simulink model "Sim5_MMC"  (R2017b)
settings: Solver=ode1  StartTime=0.0  StopTime=4  FixedStep=Time_Step  RelTol=1e-3
undefined symbols (not defined in the file): DiscIntNeverNeededParam, GRD00_Lg, GRD00_Rg, Time_Step, VSC01_id0
libraries: powerlib x107, Control_Lib x16, simulink x15, spsCurrentMeasurementLib x14, powerlib_meascontrol x4
(part 2 of 5)

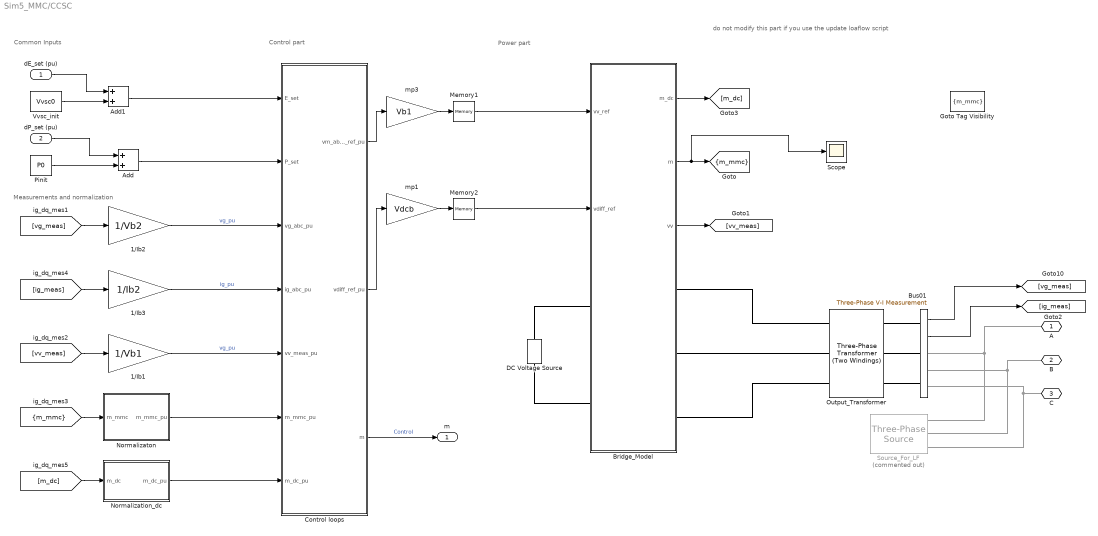
== system Sim5_MMC/CCSC ==
  note: do not modify this part if you use the update loaflow script
  note: Common Inputs
  note: Power part
  note: Measurements and normalization
  note: Control part
  dE_set (pu) : Inport
  dP_set (pu) : Inport  Port=2
  1/Ib1 : Gain  Gain=1/Vb1
  1/Ib2 : Gain  Gain=1/Vb2
  1/Ib3 : Gain  Gain=1/Ib2
  Add : Sum
  Add1 : Sum
  Bridge_Model : Subsystem
  Bus01 : powerlib/Measurements/Three-Phase V-I Measurement  VoltageMeasurement=phase-to-ground  SetLabelV=off  LabelV=Vabc  Vpu=off  VpuLL=off  CurrentMeasurement=yes  SetLabelI=off  LabelI=Iabc  Ipu=off  Pbase=100e6  Vbase=500e3  OutputType=Complex  PhasorSimulation=off  PSBequivalent=0
  Control loops : Subsystem
  DC Voltage Source : powerlib/Electrical Sources/DC Voltage Source  Amplitude=Udcn  Measurements=Voltage
  Goto Tag Visibility : GotoTagVisibility  GotoTag=m_mmc
  Memory1 : Memory  InitialCondition=[Va0 Vb0 Vc0]
  Memory2 : Memory  InitialCondition=[Udcn/2 Udcn/2 Udcn/2]
  Normalization_dc : Subsystem
  Normalizaton : Subsystem
  Output_Transformer : powerlib/Elements/Three-Phase Transformer (Two Windings)  Winding1Connection=Yg  Winding2Connection=Yg  CoreType=Three single-phase transformers  SetSaturation=off  Hysteresis=off  DataFile='hysteresis'  SetInitialFlux=off  Measurements=None  UNITS=pu  NominalPower=[Sn , fb]  Winding1=[Un1 , Rt_pu/2 , Lt_pu/2]  Winding2=[Un2 , Rt_pu/2 , Lt_pu/2]  Rm=Rm_pu  Lm=Lm_pu  L0=0.5  Saturation=[ 0,0 ; 0.0024,1.2 ; 1.0,1.52 ]  InitialFluxes=[ 0.8 , -0.8 , 0.7 ]  BreakLoop=off  DiscreteSolver=Trapezoidal iterative  DataType=off  TransfoNumber=1
  Pinit : Constant  Value=P0
  Scope : Scope
  Source_For_LF : powerlib/Electrical Sources/Three-Phase Source  Commented=on  InternalConnection=Yg  VoltagePhases=off  Voltage=(400000)*1.00095  PhaseAngle=0.57242  Voltage_phases=[25e3 25e3 25e3]/sqrt(3)  PhaseAngles_phases=[0 -120 +120]  Frequency=fb  NonIdealSource=off  SpecifyImpedance=off  Resistance=0  Inductance=0  ShortCircuitLevel=100e6  BaseVoltage=Un  XRratio=7  BusType=PQ  Pref=P0*Sb  Qref=Q0*Sb  Prefabc=[10e3, 10e3, 10e3]  Qrefabc=[0, 0, 0]  Qmin=-inf  Qmax=inf
  Vvsc_init : Constant  Value=Vvsc0
  mp1 : Gain  Gain=Vdcb
  mp3 : Gain  Gain=Vb1
  A : PMIOPort  Side=Right
  B : PMIOPort  Port=2  Side=Right
  C : PMIOPort  Port=3  Side=Right
  m : Outport  VectorParamsAs1DForOutWhenUnconnected=off
  tag scope: m_mmc=scoped
  wires:
  Add/1 -> Control loops/2(P_set)
  Control loops/3(m) -> m/1  "Control"
  mp3/1 -> Memory1/1
  1/Ib3/1 -> Control loops/4(ig_abc_pu)  "ig_pu"
  1/Ib2/1 -> Control loops/3(vg_abc_pu)  "vg_pu"
  [vg_meas] -> 1/Ib2/1
  Control loops/1(vm_abc_ref_pu) -> mp3/1
  Add1/1 -> Control loops/1(E_set)
  Memory1/1 -> Bridge_Model/1(vv_ref)
  dP_set (pu)/1 -> Add/1
  Pinit/1 -> Add/2
  Vvsc_init/1 -> Add1/2
  Bus01/1 -> [vg_meas]
  dE_set (pu)/1 -> Add1/1
  Bus01/2 -> [ig_meas]
  [ig_meas] -> 1/Ib3/1
  Control loops/2(vdiff_ref_pu) -> mp1/1
  mp1/1 -> Memory2/1
  Memory2/1 -> Bridge_Model/2(vdiff_ref)
  Bridge_Model/3(vv) -> [vv_meas]
  [vv_meas] -> 1/Ib1/1
  1/Ib1/1 -> Control loops/5(vv_meas_pu)  "vg_pu"
  [m_mmc] -> Normalizaton/1(m_mmc)
  Normalizaton/1(m_mmc_pu) -> Control loops/6(m_mmc_pu)
  Bridge_Model/1(m_dc) -> [m_dc]
  Normalization_dc/1(m_dc_pu) -> Control loops/7(m_dc_pu)
  [m_dc] -> Normalization_dc/1(m_dc)
  Bridge_Model/2(m) -> Scope/1, [m_mmc]
  connections:
  DC Voltage Source/LConn1 -- Bridge_Model/LConn2
  Output_Transformer/RConn1 -- Bus01/LConn1
  Output_Transformer/RConn2 -- Bus01/LConn2
  DC Voltage Source/RConn1 -- Bridge_Model/LConn1
  Output_Transformer/RConn3 -- Bus01/LConn3
  Source_For_LF/RConn2 -- B/RConn1 -- Bus01/RConn2
  Source_For_LF/RConn1 -- A/RConn1 -- Bus01/RConn1
  Source_For_LF/RConn3 -- C/RConn1 -- Bus01/RConn3
  Bridge_Model/RConn1 -- Output_Transformer/LConn1
  Bridge_Model/RConn2 -- Output_Transformer/LConn2
  Bridge_Model/RConn3 -- Output_Transformer/LConn3

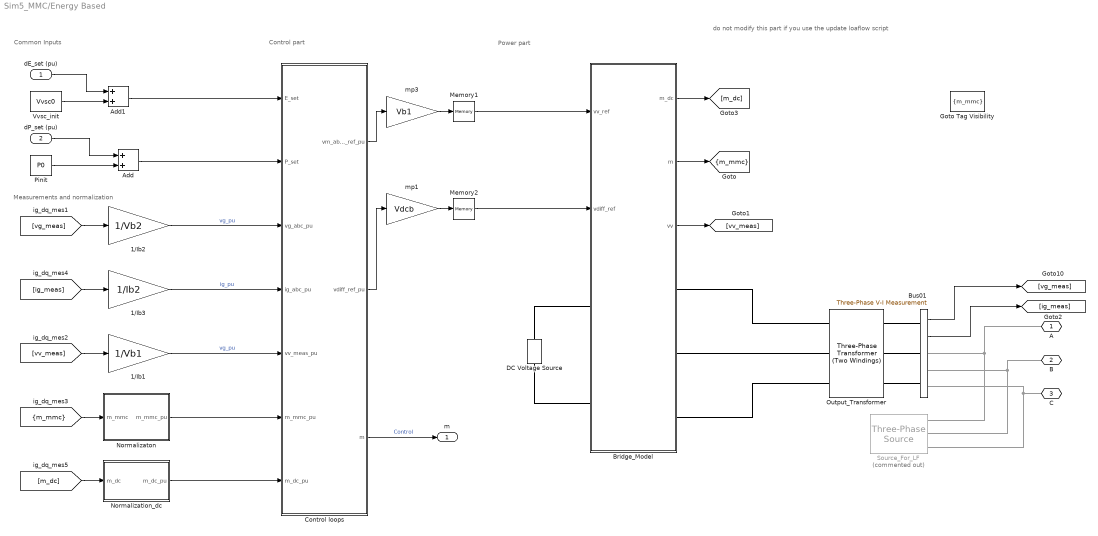
== system Sim5_MMC/Energy Based ==
  note: do not modify this part if you use the update loaflow script
  note: Common Inputs
  note: Power part
  note: Measurements and normalization
  note: Control part
  dE_set (pu) : Inport
  dP_set (pu) : Inport  Port=2
  1/Ib1 : Gain  Gain=1/Vb1
  1/Ib2 : Gain  Gain=1/Vb2
  1/Ib3 : Gain  Gain=1/Ib2
  Add : Sum
  Add1 : Sum
  Bridge_Model : Subsystem
  Bus01 : powerlib/Measurements/Three-Phase V-I Measurement  VoltageMeasurement=phase-to-ground  SetLabelV=off  LabelV=Vabc  Vpu=off  VpuLL=off  CurrentMeasurement=yes  SetLabelI=off  LabelI=Iabc  Ipu=off  Pbase=100e6  Vbase=500e3  OutputType=Complex  PhasorSimulation=off  PSBequivalent=0
  Control loops : Subsystem
  DC Voltage Source : powerlib/Electrical Sources/DC Voltage Source  Amplitude=Udcn  Measurements=Voltage
  Goto Tag Visibility : GotoTagVisibility  GotoTag=m_mmc
  Memory1 : Memory  InitialCondition=[Va0 Vb0 Vc0]
  Memory2 : Memory  InitialCondition=[Udcn/2 Udcn/2 Udcn/2]
  Normalization_dc : Subsystem
  Normalizaton : Subsystem
  Output_Transformer : powerlib/Elements/Three-Phase Transformer (Two Windings)  Winding1Connection=Yg  Winding2Connection=Yg  CoreType=Three single-phase transformers  SetSaturation=off  Hysteresis=off  DataFile='hysteresis'  SetInitialFlux=off  Measurements=None  UNITS=pu  NominalPower=[Sn , fb]  Winding1=[Un1 , Rt_pu/2 , Lt_pu/2]  Winding2=[Un2 , Rt_pu/2 , Lt_pu/2]  Rm=Rm_pu  Lm=Lm_pu  L0=0.5  Saturation=[ 0,0 ; 0.0024,1.2 ; 1.0,1.52 ]  InitialFluxes=[ 0.8 , -0.8 , 0.7 ]  BreakLoop=off  DiscreteSolver=Trapezoidal iterative  DataType=off  TransfoNumber=1
  Pinit : Constant  Value=P0
  Source_For_LF : powerlib/Electrical Sources/Three-Phase Source  Commented=on  InternalConnection=Yg  VoltagePhases=off  Voltage=(400000)*1.00095  PhaseAngle=0.57242  Voltage_phases=[25e3 25e3 25e3]/sqrt(3)  PhaseAngles_phases=[0 -120 +120]  Frequency=fb  NonIdealSource=off  SpecifyImpedance=off  Resistance=0  Inductance=0  ShortCircuitLevel=100e6  BaseVoltage=Un  XRratio=7  BusType=PQ  Pref=P0*Sb  Qref=Q0*Sb  Prefabc=[10e3, 10e3, 10e3]  Qrefabc=[0, 0, 0]  Qmin=-inf  Qmax=inf
  Vvsc_init : Constant  Value=Vvsc0
  mp1 : Gain  Gain=Vdcb
  mp3 : Gain  Gain=Vb1
  A : PMIOPort  Side=Right
  B : PMIOPort  Port=2  Side=Right
  C : PMIOPort  Port=3  Side=Right
  m : Outport  VectorParamsAs1DForOutWhenUnconnected=off
  tag scope: m_mmc=scoped
  wires:
  Add/1 -> Control loops/2(P_set)
  Control loops/3(m) -> m/1  "Control"
  mp3/1 -> Memory1/1
  1/Ib3/1 -> Control loops/4(ig_abc_pu)  "ig_pu"
  1/Ib2/1 -> Control loops/3(vg_abc_pu)  "vg_pu"
  [vg_meas] -> 1/Ib2/1
  Control loops/1(vm_abc_ref_pu) -> mp3/1
  Add1/1 -> Control loops/1(E_set)
  Memory1/1 -> Bridge_Model/1(vv_ref)
  dP_set (pu)/1 -> Add/1
  Pinit/1 -> Add/2
  Vvsc_init/1 -> Add1/2
  Bus01/1 -> [vg_meas]
  dE_set (pu)/1 -> Add1/1
  Bus01/2 -> [ig_meas]
  [ig_meas] -> 1/Ib3/1
  Control loops/2(vdiff_ref_pu) -> mp1/1
  mp1/1 -> Memory2/1
  Memory2/1 -> Bridge_Model/2(vdiff_ref)
  Bridge_Model/3(vv) -> [vv_meas]
  [vv_meas] -> 1/Ib1/1
  1/Ib1/1 -> Control loops/5(vv_meas_pu)  "vg_pu"
  [m_mmc] -> Normalizaton/1(m_mmc)
  Normalizaton/1(m_mmc_pu) -> Control loops/6(m_mmc_pu)
  Bridge_Model/1(m_dc) -> [m_dc]
  Normalization_dc/1(m_dc_pu) -> Control loops/7(m_dc_pu)
  [m_dc] -> Normalization_dc/1(m_dc)
  Bridge_Model/2(m) -> [m_mmc]
  connections:
  DC Voltage Source/LConn1 -- Bridge_Model/LConn2
  Output_Transformer/RConn1 -- Bus01/LConn1
  Output_Transformer/RConn2 -- Bus01/LConn2
  DC Voltage Source/RConn1 -- Bridge_Model/LConn1
  Output_Transformer/RConn3 -- Bus01/LConn3
  Source_For_LF/RConn2 -- B/RConn1 -- Bus01/RConn2
  Source_For_LF/RConn1 -- A/RConn1 -- Bus01/RConn1
  Source_For_LF/RConn3 -- C/RConn1 -- Bus01/RConn3
  Bridge_Model/RConn1 -- Output_Transformer/LConn1
  Bridge_Model/RConn2 -- Output_Transformer/LConn2
  Bridge_Model/RConn3 -- Output_Transformer/LConn3

== system Sim5_MMC/Mean Model 2-Level L-filter ==
  note: do not modify this part if you use the update loaflow script
  note: Common Inputs
  note: Power part
  note: Measurements and normalization
  note: Control part
  dE_set (pu) : Inport
  dP_set (pu) : Inport  Port=2
  1/Ib2 : Gain  Gain=1/Vb2
  1/Ib3 : Gain  Gain=1/Ib2
  Add : Sum
  Add1 : Sum
  Bridge_Model : Subsystem
  Bus01 : powerlib/Measurements/Three-Phase V-I Measurement  VoltageMeasurement=phase-to-ground  SetLabelV=off  LabelV=Vabc  Vpu=off  VpuLL=off  CurrentMeasurement=yes  SetLabelI=off  LabelI=Iabc  Ipu=off  Pbase=100e6  Vbase=500e3  OutputType=Complex  PhasorSimulation=off  PSBequivalent=0
  Control loops : Subsystem
  DC Voltage Source : powerlib/Electrical Sources/DC Voltage Source  Amplitude=Udcn  Measurements=Voltage
  Memory1 : Memory  InitialCondition=[Va0 Vb0 Vc0]
  Output_Transformer : powerlib/Elements/Three-Phase Transformer (Two Windings)  Winding1Connection=Yg  Winding2Connection=Yg  CoreType=Three single-phase transformers  SetSaturation=off  Hysteresis=off  DataFile='hysteresis'  SetInitialFlux=off  Measurements=None  UNITS=pu  NominalPower=[Sn , fb]  Winding1=[Un1 , Rt_pu/2 , Lt_pu/2]  Winding2=[Un2 , Rt_pu/2 , Lt_pu/2]  Rm=Rm_pu  Lm=Lm_pu  L0=0.5  Saturation=[ 0,0 ; 0.0024,1.2 ; 1.0,1.52 ]  InitialFluxes=[ 0.8 , -0.8 , 0.7 ]  BreakLoop=off  DiscreteSolver=Trapezoidal iterative  DataType=off  TransfoNumber=1
  Pinit : Constant  Value=P0
  Source_For_LF : powerlib/Electrical Sources/Three-Phase Source  Commented=on  InternalConnection=Yg  VoltagePhases=off  Voltage=(400000)*1.00139  PhaseAngle=0.85782  Voltage_phases=[25e3 25e3 25e3]/sqrt(3)  PhaseAngles_phases=[0 -120 +120]  Frequency=fb  NonIdealSource=off  SpecifyImpedance=off  Resistance=0  Inductance=0  ShortCircuitLevel=100e6  BaseVoltage=Un  XRratio=7  BusType=PQ  Pref=P0*Sb  Qref=Q0*Sb  Prefabc=[10e3, 10e3, 10e3]  Qrefabc=[0, 0, 0]  Qmin=-inf  Qmax=inf
  Vvsc_init : Constant  Value=Vvsc0
  mp3 : Gain  Gain=Vb1
  A : PMIOPort  Side=Right
  B : PMIOPort  Port=2  Side=Right
  C : PMIOPort  Port=3  Side=Right
  m : Outport  VectorParamsAs1DForOutWhenUnconnected=off
  wires:
  Add/1 -> Control loops/2(P_set)
  Control loops/2(m) -> m/1  "Control"
  mp3/1 -> Memory1/1
  1/Ib3/1 -> Control loops/4(ig_abc_pu)  "ig_pu"
  1/Ib2/1 -> Control loops/3(vg_abc_pu)  "vg_pu"
  [vg_meas] -> 1/Ib2/1
  Control loops/1(vm_abc_ref_pu) -> mp3/1
  Add1/1 -> Control loops/1(E_set)
  Memory1/1 -> Bridge_Model/1(Uref)
  dP_set (pu)/1 -> Add/1
  Pinit/1 -> Add/2
  Vvsc_init/1 -> Add1/2
  Bus01/1 -> [vg_meas]
  dE_set (pu)/1 -> Add1/1
  Bus01/2 -> [ig_meas]
  [ig_meas] -> 1/Ib3/1
  connections:
  DC Voltage Source/LConn1 -- Bridge_Model/LConn2
  Output_Transformer/RConn1 -- Bus01/LConn1
  Output_Transformer/RConn2 -- Bus01/LConn2
  DC Voltage Source/RConn1 -- Bridge_Model/LConn1
  Output_Transformer/RConn3 -- Bus01/LConn3
  Source_For_LF/RConn2 -- B/RConn1 -- Bus01/RConn2
  Bridge_Model/RConn1 -- Output_Transformer/LConn1
  Bridge_Model/RConn2 -- Output_Transformer/LConn2
  Bridge_Model/RConn3 -- Output_Transformer/LConn3
  Source_For_LF/RConn1 -- A/RConn1 -- Bus01/RConn1
  Source_For_LF/RConn3 -- C/RConn1 -- Bus01/RConn3

== system Sim5_MMC/Subsystem2 ==

== system Sim5_MMC/CCSC/Bridge_Model ==
  vv_ref : Inport
  vdiff_ref : Inport  Port=2
  Bus1 : powerlib/Measurements/Three-Phase V-I Measurement  VoltageMeasurement=phase-to-ground  SetLabelV=off  LabelV=Vabc  Vpu=off  VpuLL=off  CurrentMeasurement=no  SetLabelI=off  LabelI=Iabc  Ipu=off  Pbase=100e6  Vbase=500e3  OutputType=Complex  PhasorSimulation=off  PSBequivalent=0
  Constant : Constant
  Current Measurement : spsCurrentMeasurementLib/Current Measurement  PhasorSimulation=off  OutputType=Complex  PSBequivalent=0
  Decoupling voltage : Subsystem
  MMC Average Model : Subsystem
  Memory : Memory
  Memory1 : Memory  InitialCondition=Udcn
  Modulation Index Generation : Subsystem
  Mux : Mux  Inputs=2
  NOT1 : Logic  Operator=NOT  IconShape=distinctive  AllPortsSameDT=off  OutDataTypeStr=boolean
  Three-Phase Breaker1 : powerlib/Elements/Three-Phase Breaker  InitialState=closed  SwitchA=on  SwitchB=on  SwitchC=on  SwitchTimes="[4/60  10/60]"  External=on  BreakerResistance=0.001  SnubberResistance=1e6  SnubberCapacitance=inf  Measurements=None
  Three-Phase Breaker2 : powerlib/Elements/Three-Phase Breaker  InitialState=open  SwitchA=on  SwitchB=on  SwitchC=on  SwitchTimes="[4/60  10/60]"  External=on  BreakerResistance=0.001  SnubberResistance=1e6  SnubberCapacitance=inf  Measurements=None
  Three-Phase Source : powerlib/Electrical Sources/Three-Phase Source  InternalConnection=Yg  VoltagePhases=off  Voltage=Vvsc0*Un1  PhaseAngle=Theta_vsc0  Voltage_phases=[25e3 25e3 25e3]/sqrt(3)  PhaseAngles_phases=[0 -120 +120]  Frequency=fb  NonIdealSource=off  SpecifyImpedance=off  Resistance=0  Inductance=0  ShortCircuitLevel=100e6  BaseVoltage=VSC01_Un1  XRratio=7  BusType=swing  Pref=0.3  Qref=0  Prefabc=[10e3, 10e3, 10e3]  Qrefabc=[0, 0, 0]  Qmin=-Inf  Qmax=Inf
  Voltage Measurement : powerlib/Measurements/Voltage Measurement  PhasorSimulation=off  OutputType=Complex  PSBequivalent=0
  PhA : PMIOPort  Side=Right
  PhB : PMIOPort  Port=2  Side=Right
  PhC : PMIOPort  Port=3  Side=Right
  Vdc+ : PMIOPort  Port=4  Side=Left
  Vdc- : PMIOPort  Port=5  Side=Left
  m_dc : Outport
  m : Outport  Port=2
  vv : Outport  Port=3
  wires:
  Constant/1 -> Memory/1
  NOT1/1 -> Three-Phase Breaker1/1
  Memory/1 -> NOT1/1, Three-Phase Breaker2/1
  vv_ref/1 -> Decoupling voltage/1(Vv_ref)
  vdiff_ref/1 -> Decoupling voltage/2(Vdiff_ref)
  Decoupling voltage/1(Vmu_ref) -> Modulation Index Generation/1(vmu_ref)
  Decoupling voltage/2(Vml_ref) -> Modulation Index Generation/2(vml_ref)
  MMC Average Model/1(m) -> m/1
  Voltage Measurement/1 -> Memory1/1  "Vdc"
  Current Measurement/1 -> Mux/2  "Idc"
  Mux/1 -> m_dc/1
  Modulation Index Generation/1(mul) -> MMC Average Model/1(mul)
  Bus1/1 -> vv/1
  Memory1/1 -> Mux/1
  connections:
  Three-Phase Breaker1/LConn1 -- Bus1/LConn1 -- Three-Phase Breaker2/LConn1
  Three-Phase Breaker1/LConn2 -- Bus1/LConn2 -- Three-Phase Breaker2/LConn2
  Three-Phase Breaker1/LConn3 -- Bus1/LConn3 -- Three-Phase Breaker2/LConn3
  MMC Average Model/LConn1 -- Three-Phase Breaker2/RConn1
  MMC Average Model/LConn2 -- Three-Phase Breaker2/RConn2
  MMC Average Model/LConn3 -- Three-Phase Breaker2/RConn3
  Three-Phase Source/RConn1 -- Three-Phase Breaker1/RConn1
  Three-Phase Source/RConn2 -- Three-Phase Breaker1/RConn2
  Three-Phase Source/RConn3 -- Three-Phase Breaker1/RConn3
  MMC Average Model/RConn1 -- Current Measurement/RConn1 -- Voltage Measurement/LConn1
  MMC Average Model/RConn2 -- Voltage Measurement/LConn2 -- Vdc-/RConn1
  Current Measurement/LConn1 -- Vdc+/RConn1
  PhB/RConn1 -- Bus1/RConn2
  PhC/RConn1 -- Bus1/RConn3
  PhA/RConn1 -- Bus1/RConn1

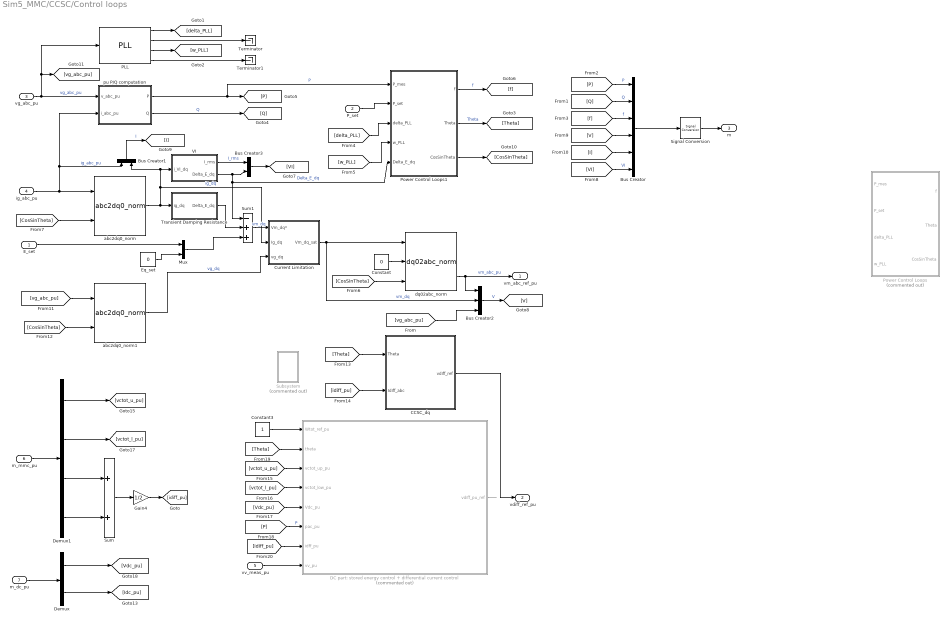
== system Sim5_MMC/CCSC/Control loops ==
  E_set : Inport
  P_set : Inport  Port=2
  vg_abc_pu : Inport  Port=3
  ig_abc_pu : Inport  Port=4
  vv_meas_pu : Inport  Port=5
  m_mmc_pu : Inport  Port=6
  m_dc_pu : Inport  Port=7
  " pu P/Q computation" : Subsystem  DialogController=POWERSYS.PowerSysDialog
  Bus Creator : BusCreator  Inputs=6
  Bus Creator1 : BusCreator  Inputs=2
  Bus Creator2 : BusCreator  Inputs=3
  Bus Creator3 : BusCreator  Inputs=2
  CCSC_dq : Subsystem
  Constant : Constant  Value=0
  Constant3 : Constant
  Current Limitation : Subsystem
  DC part: stored energy control + differential current control : Subsystem  Commented=on
  Demux : Demux  Outputs=2
  Demux1 : Demux  Outputs=[3 3 3 3]
  Eq_set : Constant  Value=0
  Gain4 : Gain  Gain=1/2
  Mux : Mux  Inputs=2
  PLL : Control_Lib/PLL  fb=fb  Tr_PLL=Tr_PLL  Theta0=Theta0
      settings: SourceProductName=VSC_Lib
  Power Control Loops : Subsystem  Commented=on
  Power Control Loops1 : Subsystem
  Signal Conversion : SignalConversion  OverrideOpt=off
  Subsystem : Subsystem  Commented=on
  Sum : Sum
  Sum1 : Sum  Inputs=-++
  Terminator : Terminator
  Terminator1 : Terminator
  Transient Damping Resistance : Subsystem
  VI : Subsystem
  abc2dq0_norm : Control_Lib/abc2dq0_norm  referenceAxisMode=Reference axis at 90 degrees behind phase_a  baseUpdateGain=1/sqrt(3)
      settings: SourceProductName=VSC_Lib
  abc2dq0_norm1 : Control_Lib/abc2dq0_norm  referenceAxisMode=Reference axis at 90 degrees behind phase_a  baseUpdateGain=1/sqrt(3)
      settings: SourceProductName=VSC_Lib
  dq02abc_norm : Control_Lib/dq02abc_norm  referenceAxisMode=Reference axis at 90 degrees behind phase_a  baseUpdateGain=sqrt(3)
      settings: SourceProductName=VSC_Lib
  vm_abc_ref_pu : Outport  VectorParamsAs1DForOutWhenUnconnected=off
  vdiff_ref_pu : Outport  Port=2
  m : Outport  Port=3  VectorParamsAs1DForOutWhenUnconnected=off
  wires:
  [vg_abc_pu] -> Bus Creator2/3
  Bus Creator3/1 -> [VI]
  PLL/4 -> Terminator1/1
  PLL/2 -> Terminator/1
  PLL/1 -> [delta_PLL]
  Constant/1 -> dq02abc_norm/2
  Power Control Loops1/3(CosSinTheta) -> [CosSinTheta]
  PLL/3 -> [w_PLL]
  [I] -> Bus Creator/5
  Bus Creator1/1 -> [I]  "I"
  Bus Creator/1 -> Signal Conversion/1
  [VI] -> Bus Creator/6  "VI"
  [V] -> Bus Creator/4
  Bus Creator2/1 -> [V]  "V"
  Eq_set/1 -> Mux/2
  Mux/1 -> Sum1/3
  VI/1(I_rms) -> Bus Creator3/1  "I_rms"
  Transient Damping Resistance/1("Delta_E_dq ") -> Sum1/2
  VI/2(Delta_E_dq) -> Power Control Loops1/5(Delta_E_dq), Sum1/1, Bus Creator3/2  "Delta_E_dq"
  [CosSinTheta] -> abc2dq0_norm/2
  [CosSinTheta] -> dq02abc_norm/3
  Power Control Loops1/2(Theta) -> [Theta]  "Theta"
  abc2dq0_norm/2 -> Bus Creator1/2, VI/1(i_VI_dq), Current Limitation/2(Ig_dq), Transient Damping Resistance/1(ig_dq)  "ig_dq"
  ig_abc_pu/1 -> abc2dq0_norm/1, " pu P/Q computation"/2(i_abc_pu), Bus Creator1/1  "ig_abc_pu"
  " pu P/Q computation"/1(P) -> Power Control Loops1/1(P_mes), [P]  "P"
  vg_abc_pu/1 -> PLL/1, [vg_abc_pu], " pu P/Q computation"/1(v_abc_pu)  "vg_abc_pu"
  Power Control Loops1/1(f) -> [f]  "f"
  [w_PLL] -> Power Control Loops1/4(w_PLL)
  P_set/1 -> Power Control Loops1/2(P_set)
  [delta_PLL] -> Power Control Loops1/3(delta_PLL)
  Current Limitation/1(Vm_dq_sat) -> dq02abc_norm/1, Bus Creator2/2  "vm_dq"
  " pu P/Q computation"/2(Q) -> [Q]  "Q"
  E_set/1 -> Mux/1
  dq02abc_norm/2 -> vm_abc_ref_pu/1, Bus Creator2/1  "vm_abc_pu"
  [f] -> Bus Creator/3  "f"
  [Q] -> Bus Creator/2  "Q"
  [P] -> Bus Creator/1  "P"
  Signal Conversion/1 -> m/1
  Sum1/1 -> Current Limitation/1(Vm_dq*)  "vm_dq"
  [vg_abc_pu] -> abc2dq0_norm1/1
  [CosSinTheta] -> abc2dq0_norm1/2
  abc2dq0_norm1/2 -> Current Limitation/3(vg_dq)  "vg_dq"
  [idiff_pu] -> CCSC_dq/2(Idiff_abc)
  CCSC_dq/1(vdiff_ref) -> vdiff_ref_pu/1
  Demux1/2 -> [vctot_l_pu]
  Demux1/1 -> [vctot_u_pu]
  m_mmc_pu/1 -> Demux1/1
  Demux/2 -> [Idc_pu]
  Demux/1 -> [Vdc_pu]
  m_dc_pu/1 -> Demux/1
  [Theta] -> CCSC_dq/1(Theta)
  Gain4/1 -> [idiff_pu]
  Sum/1 -> Gain4/1
  Demux1/3 -> Sum/1
  Demux1/4 -> Sum/2
  [vctot_u_pu] -> DC part: stored energy control + differential current control/3(vctot_up_pu)
  [vctot_l_pu] -> DC part: stored energy control + differential current control/4(vctot_low_pu)
  [Vdc_pu] -> DC part: stored energy control + differential current control/5(Vdc_pu)
  [P] -> DC part: stored energy control + differential current control/6(pac_pu)  "P"
  Constant3/1 -> DC part: stored energy control + differential current control/1(Wtot_ref_pu)
  [Theta] -> DC part: stored energy control + differential current control/2(theta)
  [idiff_pu] -> DC part: stored energy control + differential current control/7(idff_pu)
  DC part: stored energy control + differential current control/1(vdiff_pu_ref) -> ?
  vv_meas_pu/1 -> DC part: stored energy control + differential current control/8(vv_pu)

== system Sim5_MMC/CCSC/Normalization_dc ==
  m_dc : Inport
  Demux : Demux  Outputs=2
  Gain11 : Gain  Gain=1/Vdcb
  Gain12 : Gain  Gain=1/Idcb
  Mux : Mux  Inputs=2
  m_dc_pu : Outport
  wires:
  Mux/1 -> m_dc_pu/1
  Demux/2 -> Gain12/1
  Gain12/1 -> Mux/2  "Idc_pu"
  Gain11/1 -> Mux/1  "Vdc_pu"
  Demux/1 -> Gain11/1
  m_dc/1 -> Demux/1

== system Sim5_MMC/CCSC/Normalizaton ==
  m_mmc : Inport
  Demux : Demux  Outputs=[3 3 3 3]
  Gain : Gain  Gain=1/Idcb
  Gain3 : Gain  Gain=1/Idcb
  Gain6 : Gain  Gain=1/Vdcb
  Gain8 : Gain  Gain=1/Vdcb
  Mux : Mux
  m_mmc_pu : Outport
  wires:
  m_mmc/1 -> Demux/1
  Mux/1 -> m_mmc_pu/1
  Demux/3 -> Gain/1
  Gain/1 -> Mux/3  "i_arm_u_pu"
  Demux/4 -> Gain3/1
  Gain3/1 -> Mux/4  "i_arm_l_pu"
  Demux/2 -> Gain8/1
  Gain6/1 -> Mux/1  "vctot_u_pu"
  Demux/1 -> Gain6/1
  Gain8/1 -> Mux/2  "vctot_l_pu"

== system Sim5_MMC/Energy Based/Bridge_Model ==
  vv_ref : Inport
  vdiff_ref : Inport  Port=2
  Bus1 : powerlib/Measurements/Three-Phase V-I Measurement  VoltageMeasurement=phase-to-ground  SetLabelV=off  LabelV=Vabc  Vpu=off  VpuLL=off  CurrentMeasurement=no  SetLabelI=off  LabelI=Iabc  Ipu=off  Pbase=100e6  Vbase=500e3  OutputType=Complex  PhasorSimulation=off  PSBequivalent=0
  Constant : Constant
  Current Measurement : spsCurrentMeasurementLib/Current Measurement  PhasorSimulation=off  OutputType=Complex  PSBequivalent=0
  Decoupling voltage : Subsystem
  MMC Average Model : Subsystem
  Memory : Memory
  Memory1 : Memory  InitialCondition=Udcn
  Modulation Index Generation : Subsystem
  Mux : Mux  Inputs=2
  NOT1 : Logic  Operator=NOT  IconShape=distinctive  AllPortsSameDT=off  OutDataTypeStr=boolean
  Three-Phase Breaker1 : powerlib/Elements/Three-Phase Breaker  InitialState=closed  SwitchA=on  SwitchB=on  SwitchC=on  SwitchTimes="[4/60  10/60]"  External=on  BreakerResistance=0.001  SnubberResistance=1e6  SnubberCapacitance=inf  Measurements=None
  Three-Phase Breaker2 : powerlib/Elements/Three-Phase Breaker  InitialState=open  SwitchA=on  SwitchB=on  SwitchC=on  SwitchTimes="[4/60  10/60]"  External=on  BreakerResistance=0.001  SnubberResistance=1e6  SnubberCapacitance=inf  Measurements=None
  Three-Phase Source : powerlib/Electrical Sources/Three-Phase Source  InternalConnection=Yg  VoltagePhases=off  Voltage=Vvsc0*Un1  PhaseAngle=Theta_vsc0  Voltage_phases=[25e3 25e3 25e3]/sqrt(3)  PhaseAngles_phases=[0 -120 +120]  Frequency=fb  NonIdealSource=off  SpecifyImpedance=off  Resistance=0  Inductance=0  ShortCircuitLevel=100e6  BaseVoltage=VSC01_Un1  XRratio=7  BusType=swing  Pref=0.3  Qref=0  Prefabc=[10e3, 10e3, 10e3]  Qrefabc=[0, 0, 0]  Qmin=-Inf  Qmax=Inf
  Voltage Measurement : powerlib/Measurements/Voltage Measurement  PhasorSimulation=off  OutputType=Complex  PSBequivalent=0
  PhA : PMIOPort  Side=Right
  PhB : PMIOPort  Port=2  Side=Right
  PhC : PMIOPort  Port=3  Side=Right
  Vdc+ : PMIOPort  Port=4  Side=Left
  Vdc- : PMIOPort  Port=5  Side=Left
  m_dc : Outport
  m : Outport  Port=2
  vv : Outport  Port=3
  wires:
  Constant/1 -> Memory/1
  NOT1/1 -> Three-Phase Breaker1/1
  Memory/1 -> NOT1/1, Three-Phase Breaker2/1
  vv_ref/1 -> Decoupling voltage/1(Vv_ref)
  vdiff_ref/1 -> Decoupling voltage/2(Vdiff_ref)
  Decoupling voltage/1(Vmu_ref) -> Modulation Index Generation/1(vmu_ref)
  Decoupling voltage/2(Vml_ref) -> Modulation Index Generation/2(vml_ref)
  MMC Average Model/1(m) -> m/1
  Voltage Measurement/1 -> Memory1/1  "Vdc"
  Current Measurement/1 -> Mux/2  "Idc"
  Mux/1 -> m_dc/1
  Modulation Index Generation/1(mul) -> MMC Average Model/1(mul)
  Bus1/1 -> vv/1
  Memory1/1 -> Mux/1
  connections:
  Three-Phase Breaker1/LConn1 -- Bus1/LConn1 -- Three-Phase Breaker2/LConn1
  Three-Phase Breaker1/LConn2 -- Bus1/LConn2 -- Three-Phase Breaker2/LConn2
  Three-Phase Breaker1/LConn3 -- Bus1/LConn3 -- Three-Phase Breaker2/LConn3
  MMC Average Model/LConn1 -- Three-Phase Breaker2/RConn1
  MMC Average Model/LConn2 -- Three-Phase Breaker2/RConn2
  MMC Average Model/LConn3 -- Three-Phase Breaker2/RConn3
  Three-Phase Source/RConn1 -- Three-Phase Breaker1/RConn1
  Three-Phase Source/RConn2 -- Three-Phase Breaker1/RConn2
  Three-Phase Source/RConn3 -- Three-Phase Breaker1/RConn3
  MMC Average Model/RConn1 -- Current Measurement/RConn1 -- Voltage Measurement/LConn1
  MMC Average Model/RConn2 -- Voltage Measurement/LConn2 -- Vdc-/RConn1
  Current Measurement/LConn1 -- Vdc+/RConn1
  PhB/RConn1 -- Bus1/RConn2
  PhC/RConn1 -- Bus1/RConn3
  PhA/RConn1 -- Bus1/RConn1

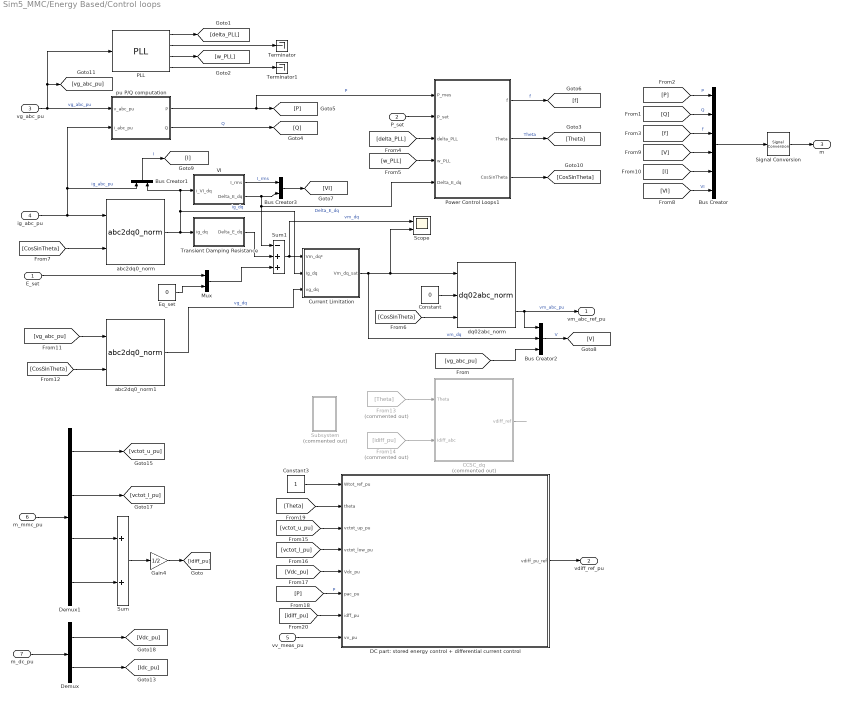
== system Sim5_MMC/Energy Based/Control loops ==
  E_set : Inport
  P_set : Inport  Port=2
  vg_abc_pu : Inport  Port=3
  ig_abc_pu : Inport  Port=4
  vv_meas_pu : Inport  Port=5
  m_mmc_pu : Inport  Port=6
  m_dc_pu : Inport  Port=7
  " pu P/Q computation" : Subsystem  DialogController=POWERSYS.PowerSysDialog
  Bus Creator : BusCreator  Inputs=6
  Bus Creator1 : BusCreator  Inputs=2
  Bus Creator2 : BusCreator  Inputs=3
  Bus Creator3 : BusCreator  Inputs=2
  CCSC_dq : Subsystem  Commented=on
  Constant : Constant  Value=0
  Constant3 : Constant
  Current Limitation : Subsystem
  DC part: stored energy control + differential current control : Subsystem
  Demux : Demux  Outputs=2
  Demux1 : Demux  Outputs=[3 3 3 3]
  Eq_set : Constant  Value=0
  From13 : From  Commented=on  GotoTag=Theta
  From14 : From  Commented=on  GotoTag=idiff_pu
  Gain4 : Gain  Gain=1/2
  Mux : Mux  Inputs=2
  PLL : Control_Lib/PLL  fb=fb  Tr_PLL=Tr_PLL  Theta0=Theta0
      settings: SourceProductName=VSC_Lib
  Power Control Loops1 : Subsystem
  Scope : Scope  NumInputPorts=2
  Signal Conversion : SignalConversion  OverrideOpt=off
  Subsystem : Subsystem  Commented=on
  Sum : Sum
  Sum1 : Sum  Inputs=-++
  Terminator : Terminator
  Terminator1 : Terminator
  Transient Damping Resistance : Subsystem
  VI : Subsystem
  abc2dq0_norm : Control_Lib/abc2dq0_norm  referenceAxisMode=Reference axis at 90 degrees behind phase_a  baseUpdateGain=1/sqrt(3)
      settings: SourceProductName=VSC_Lib
  abc2dq0_norm1 : Control_Lib/abc2dq0_norm  referenceAxisMode=Reference axis at 90 degrees behind phase_a  baseUpdateGain=1/sqrt(3)
      settings: SourceProductName=VSC_Lib
  dq02abc_norm : Control_Lib/dq02abc_norm  referenceAxisMode=Reference axis at 90 degrees behind phase_a  baseUpdateGain=sqrt(3)
      settings: SourceProductName=VSC_Lib
  vm_abc_ref_pu : Outport  VectorParamsAs1DForOutWhenUnconnected=off
  vdiff_ref_pu : Outport  Port=2
  m : Outport  Port=3  VectorParamsAs1DForOutWhenUnconnected=off
  wires:
  [vg_abc_pu] -> Bus Creator2/3
  Bus Creator3/1 -> [VI]
  PLL/4 -> Terminator1/1
  PLL/2 -> Terminator/1
  PLL/1 -> [delta_PLL]
  Constant/1 -> dq02abc_norm/2
  Power Control Loops1/3(CosSinTheta) -> [CosSinTheta]
  PLL/3 -> [w_PLL]
  [I] -> Bus Creator/5
  Bus Creator1/1 -> [I]  "I"
  Bus Creator/1 -> Signal Conversion/1
  [VI] -> Bus Creator/6  "VI"
  [V] -> Bus Creator/4
  Bus Creator2/1 -> [V]  "V"
  Eq_set/1 -> Mux/2
  Mux/1 -> Sum1/3
  VI/1(I_rms) -> Bus Creator3/1  "I_rms"
  Transient Damping Resistance/1("Delta_E_dq ") -> Sum1/2
  VI/2(Delta_E_dq) -> Power Control Loops1/5(Delta_E_dq), Sum1/1, Bus Creator3/2  "Delta_E_dq"
  [CosSinTheta] -> abc2dq0_norm/2
  [CosSinTheta] -> dq02abc_norm/3
  Power Control Loops1/2(Theta) -> [Theta]  "Theta"
  abc2dq0_norm/2 -> Bus Creator1/2, VI/1(i_VI_dq), Current Limitation/2(Ig_dq), Transient Damping Resistance/1(ig_dq)  "ig_dq"
  ig_abc_pu/1 -> abc2dq0_norm/1, " pu P/Q computation"/2(i_abc_pu), Bus Creator1/1  "ig_abc_pu"
  " pu P/Q computation"/1(P) -> Power Control Loops1/1(P_mes), [P]  "P"
  vg_abc_pu/1 -> PLL/1, [vg_abc_pu], " pu P/Q computation"/1(v_abc_pu)  "vg_abc_pu"
  Power Control Loops1/1(f) -> [f]  "f"
  P_set/1 -> Power Control Loops1/2(P_set)
  [delta_PLL] -> Power Control Loops1/3(delta_PLL)
  Current Limitation/1(Vm_dq_sat) -> Scope/2, dq02abc_norm/1, Bus Creator2/2  "vm_dq"
  " pu P/Q computation"/2(Q) -> [Q]  "Q"
  E_set/1 -> Mux/1
  dq02abc_norm/2 -> vm_abc_ref_pu/1, Bus Creator2/1  "vm_abc_pu"
  [f] -> Bus Creator/3  "f"
  [Q] -> Bus Creator/2  "Q"
  [P] -> Bus Creator/1  "P"
  Signal Conversion/1 -> m/1
  Sum1/1 -> Scope/1, Current Limitation/1(Vm_dq*)  "vm_dq"
  [vg_abc_pu] -> abc2dq0_norm1/1
  [CosSinTheta] -> abc2dq0_norm1/2
  abc2dq0_norm1/2 -> Current Limitation/3(vg_dq)  "vg_dq"
  From14/1 -> CCSC_dq/2(Idiff_abc)
  CCSC_dq/1(vdiff_ref) -> ?
  Demux1/2 -> [vctot_l_pu]
  Demux1/1 -> [vctot_u_pu]
  m_mmc_pu/1 -> Demux1/1
  Demux/2 -> [Idc_pu]
  Demux/1 -> [Vdc_pu]
  m_dc_pu/1 -> Demux/1
  From13/1 -> CCSC_dq/1(Theta)
  Gain4/1 -> [idiff_pu]
  Sum/1 -> Gain4/1
  Demux1/3 -> Sum/1
  Demux1/4 -> Sum/2
  [vctot_u_pu] -> DC part: stored energy control + differential current control/3(vctot_up_pu)
  [vctot_l_pu] -> DC part: stored energy control + differential current control/4(vctot_low_pu)
  [Vdc_pu] -> DC part: stored energy control + differential current control/5(Vdc_pu)
  [P] -> DC part: stored energy control + differential current control/6(pac_pu)  "P"
  Constant3/1 -> DC part: stored energy control + differential current control/1(Wtot_ref_pu)
  [Theta] -> DC part: stored energy control + differential current control/2(theta)
  [idiff_pu] -> DC part: stored energy control + differential current control/7(idff_pu)
  DC part: stored energy control + differential current control/1(vdiff_pu_ref) -> vdiff_ref_pu/1
  vv_meas_pu/1 -> DC part: stored energy control + differential current control/8(vv_pu)
  [w_PLL] -> Power Control Loops1/4(w_PLL)

== system Sim5_MMC/Energy Based/Normalization_dc ==
  m_dc : Inport
  Demux : Demux  Outputs=2
  Gain11 : Gain  Gain=1/Vdcb
  Gain12 : Gain  Gain=1/Idcb
  Mux : Mux  Inputs=2
  m_dc_pu : Outport
  wires:
  Mux/1 -> m_dc_pu/1
  Demux/2 -> Gain12/1
  Gain12/1 -> Mux/2  "Idc_pu"
  Gain11/1 -> Mux/1  "Vdc_pu"
  Demux/1 -> Gain11/1
  m_dc/1 -> Demux/1

== system Sim5_MMC/Energy Based/Normalizaton ==
  m_mmc : Inport
  Demux : Demux  Outputs=[3 3 3 3]
  Gain : Gain  Gain=1/Idcb
  Gain3 : Gain  Gain=1/Idcb
  Gain6 : Gain  Gain=1/Vdcb
  Gain8 : Gain  Gain=1/Vdcb
  Mux : Mux
  m_mmc_pu : Outport
  wires:
  m_mmc/1 -> Demux/1
  Mux/1 -> m_mmc_pu/1
  Demux/3 -> Gain/1
  Gain/1 -> Mux/3  "i_arm_u_pu"
  Demux/4 -> Gain3/1
  Gain3/1 -> Mux/4  "i_arm_l_pu"
  Demux/2 -> Gain8/1
  Gain6/1 -> Mux/1  "vctot_u_pu"
  Demux/1 -> Gain6/1
  Gain8/1 -> Mux/2  "vctot_l_pu"

== system Sim5_MMC/Mean Model 2-Level L-filter/Bridge_Model ==
  Uref : Inport
  Constant : Constant
  Memory : Memory
  NOT1 : Logic  Operator=NOT  IconShape=distinctive  AllPortsSameDT=off  OutDataTypeStr=boolean
  Saturation : Saturate  UpperLimit=1  LowerLimit=-1
  Three-Phase Breaker1 : powerlib/Elements/Three-Phase Breaker  InitialState=closed  SwitchA=on  SwitchB=on  SwitchC=on  SwitchTimes="[4/60  10/60]"  External=on  BreakerResistance=0.001  SnubberResistance=1e6  SnubberCapacitance=inf  Measurements=None
  Three-Phase Breaker2 : powerlib/Elements/Three-Phase Breaker  InitialState=open  SwitchA=on  SwitchB=on  SwitchC=on  SwitchTimes="[4/60  10/60]"  External=on  BreakerResistance=0.001  SnubberResistance=1e6  SnubberCapacitance=inf  Measurements=None
  Three-Phase Source : powerlib/Electrical Sources/Three-Phase Source  InternalConnection=Yg  VoltagePhases=off  Voltage=Vvsc0*Un1  PhaseAngle=Theta_vsc0  Voltage_phases=[25e3 25e3 25e3]/sqrt(3)  PhaseAngles_phases=[0 -120 +120]  Frequency=fb  NonIdealSource=off  SpecifyImpedance=off  Resistance=0  Inductance=0  ShortCircuitLevel=100e6  BaseVoltage=VSC01_Un1  XRratio=7  BusType=swing  Pref=0.3  Qref=0  Prefabc=[10e3, 10e3, 10e3]  Qrefabc=[0, 0, 0]  Qmin=-Inf  Qmax=Inf
  Universal Bridge : powerlib/Power Electronics/Universal Bridge  Arms=3  SnubberResistance=1e5  SnubberCapacitance=inf  Device=Average-model based VSC  Ron=1e-3  Lon=0  ForwardVoltages="[  0  0  ]"  ForwardVoltage=0  GTOparameters=[ 10e-6 , 20e-6 ]  IGBTparameters=[ 1e-6 , 2e-6 ]  Measurements=None  Measurements_2=None  converterType=Rectifier
  mp3 : Gain  Gain=2/Udcn
  PhA : PMIOPort  Side=Right
  PhB : PMIOPort  Port=2  Side=Right
  PhC : PMIOPort  Port=3  Side=Right
  Vdc+ : PMIOPort  Port=4  Side=Left
  Vdc- : PMIOPort  Port=5  Side=Left
  wires:
  Saturation/1 -> Universal Bridge/1
  Constant/1 -> Memory/1
  NOT1/1 -> Three-Phase Breaker1/1
  Memory/1 -> NOT1/1, Three-Phase Breaker2/1
  mp3/1 -> Saturation/1
  Uref/1 -> mp3/1
  connections:
  Three-Phase Breaker2/LConn1 -- Three-Phase Breaker1/LConn1 -- PhA/RConn1
  Three-Phase Breaker2/LConn2 -- Three-Phase Breaker1/LConn2 -- PhB/RConn1
  Three-Phase Breaker2/LConn3 -- Three-Phase Breaker1/LConn3 -- PhC/RConn1
  Three-Phase Breaker2/RConn1 -- Universal Bridge/LConn1
  Three-Phase Breaker2/RConn2 -- Universal Bridge/LConn2
  Three-Phase Breaker2/RConn3 -- Universal Bridge/LConn3
  Three-Phase Source/RConn1 -- Three-Phase Breaker1/RConn1
  Three-Phase Source/RConn2 -- Three-Phase Breaker1/RConn2
  Three-Phase Source/RConn3 -- Three-Phase Breaker1/RConn3
  Universal Bridge/RConn1 -- Vdc+/RConn1
  Universal Bridge/RConn2 -- Vdc-/RConn1

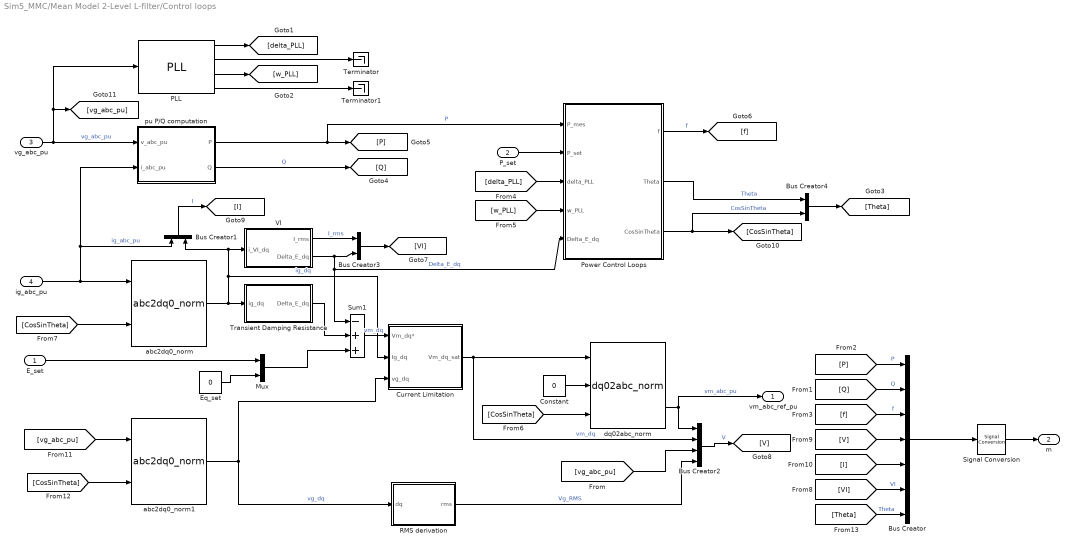
== system Sim5_MMC/Mean Model 2-Level L-filter/Control loops ==
  E_set : Inport
  P_set : Inport  Port=2
  vg_abc_pu : Inport  Port=3
  ig_abc_pu : Inport  Port=4
  " pu P/Q computation" : Subsystem  DialogController=POWERSYS.PowerSysDialog
  Bus Creator : BusCreator  Inputs=7
  Bus Creator1 : BusCreator  Inputs=2
  Bus Creator2 : BusCreator  Inputs=4
  Bus Creator3 : BusCreator  Inputs=2
  Bus Creator4 : BusCreator  Inputs=2
  Constant : Constant  Value=0
  Current Limitation : Subsystem
  Eq_set : Constant  Value=0
  Mux : Mux  Inputs=2
  PLL : Control_Lib/PLL  fb=fb  Tr_PLL=Tr_PLL  Theta0=Theta0
      settings: SourceProductName=VSC_Lib
  Power Control Loops : Subsystem
  RMS derivation : Subsystem
  Signal Conversion : SignalConversion  OverrideOpt=off
  Sum1 : Sum  Inputs=-++
  Terminator : Terminator
  Terminator1 : Terminator
  Transient Damping Resistance : Subsystem
  VI : Subsystem
  abc2dq0_norm : Control_Lib/abc2dq0_norm  referenceAxisMode=Reference axis at 90 degrees behind phase_a  baseUpdateGain=1/sqrt(3)
      settings: SourceProductName=VSC_Lib
  abc2dq0_norm1 : Control_Lib/abc2dq0_norm  referenceAxisMode=Reference axis at 90 degrees behind phase_a  baseUpdateGain=1/sqrt(3)
      settings: SourceProductName=VSC_Lib
  dq02abc_norm : Control_Lib/dq02abc_norm  referenceAxisMode=Reference axis at 90 degrees behind phase_a  baseUpdateGain=sqrt(3)
      settings: SourceProductName=VSC_Lib
  vm_abc_ref_pu : Outport  VectorParamsAs1DForOutWhenUnconnected=off
  m : Outport  Port=2  VectorParamsAs1DForOutWhenUnconnected=off
  wires:
  [Theta] -> Bus Creator/7  "Theta"
  Bus Creator4/1 -> [Theta]
  RMS derivation/1(rms) -> Bus Creator2/4  "Vg_RMS"
  [vg_abc_pu] -> Bus Creator2/3
  Bus Creator3/1 -> [VI]
  PLL/4 -> Terminator1/1
  PLL/2 -> Terminator/1
  PLL/1 -> [delta_PLL]
  Constant/1 -> dq02abc_norm/2
  Power Control Loops/3(CosSinTheta) -> [CosSinTheta], Bus Creator4/2  "CosSinTheta"
  PLL/3 -> [w_PLL]
  [I] -> Bus Creator/5
  Bus Creator1/1 -> [I]  "I"
  Bus Creator/1 -> Signal Conversion/1
  [VI] -> Bus Creator/6  "VI"
  [V] -> Bus Creator/4
  Bus Creator2/1 -> [V]  "V"
  Eq_set/1 -> Mux/2
  Mux/1 -> Sum1/3
  VI/1(I_rms) -> Bus Creator3/1  "I_rms"
  Transient Damping Resistance/1("Delta_E_dq ") -> Sum1/2
  VI/2(Delta_E_dq) -> Bus Creator3/2, Sum1/1, Power Control Loops/5(Delta_E_dq)  "Delta_E_dq"
  [CosSinTheta] -> abc2dq0_norm/2
  [CosSinTheta] -> dq02abc_norm/3
  Power Control Loops/2(Theta) -> Bus Creator4/1  "Theta"
  abc2dq0_norm/2 -> Bus Creator1/2, VI/1(i_VI_dq), Current Limitation/2(Ig_dq), Transient Damping Resistance/1(ig_dq)  "ig_dq"
  ig_abc_pu/1 -> abc2dq0_norm/1, " pu P/Q computation"/2(i_abc_pu), Bus Creator1/1  "ig_abc_pu"
  " pu P/Q computation"/1(P) -> [P], Power Control Loops/1(P_mes)  "P"
  vg_abc_pu/1 -> PLL/1, [vg_abc_pu], " pu P/Q computation"/1(v_abc_pu)  "vg_abc_pu"
  Power Control Loops/1(f) -> [f]  "f"
  [w_PLL] -> Power Control Loops/4(w_PLL)
  P_set/1 -> Power Control Loops/2(P_set)
  [delta_PLL] -> Power Control Loops/3(delta_PLL)
  Current Limitation/1(Vm_dq_sat) -> dq02abc_norm/1, Bus Creator2/2  "vm_dq"
  " pu P/Q computation"/2(Q) -> [Q]  "Q"
  E_set/1 -> Mux/1
  dq02abc_norm/2 -> Bus Creator2/1, vm_abc_ref_pu/1  "vm_abc_pu"
  [f] -> Bus Creator/3  "f"
  [Q] -> Bus Creator/2  "Q"
  [P] -> Bus Creator/1  "P"
  Signal Conversion/1 -> m/1
  Sum1/1 -> Current Limitation/1(Vm_dq*)  "vm_dq"
  [vg_abc_pu] -> abc2dq0_norm1/1
  [CosSinTheta] -> abc2dq0_norm1/2
  abc2dq0_norm1/2 -> Current Limitation/3(vg_dq), RMS derivation/1(dq)  "vg_dq"

== system Sim5_MMC/CCSC/Bridge_Model/Decoupling voltage ==
  Vv_ref : Inport
  Vdiff_ref : Inport  Port=2
  Sum7 : Sum  Inputs=+-
  Sum8 : Sum
  Vmu_ref : Outport
  Vml_ref : Outport  Port=2
  wires:
  Sum8/1 -> Vml_ref/1  "Ul"
  Sum7/1 -> Vmu_ref/1
  Vdiff_ref/1 -> Sum8/1, Sum7/1
  Vv_ref/1 -> Sum8/2, Sum7/2

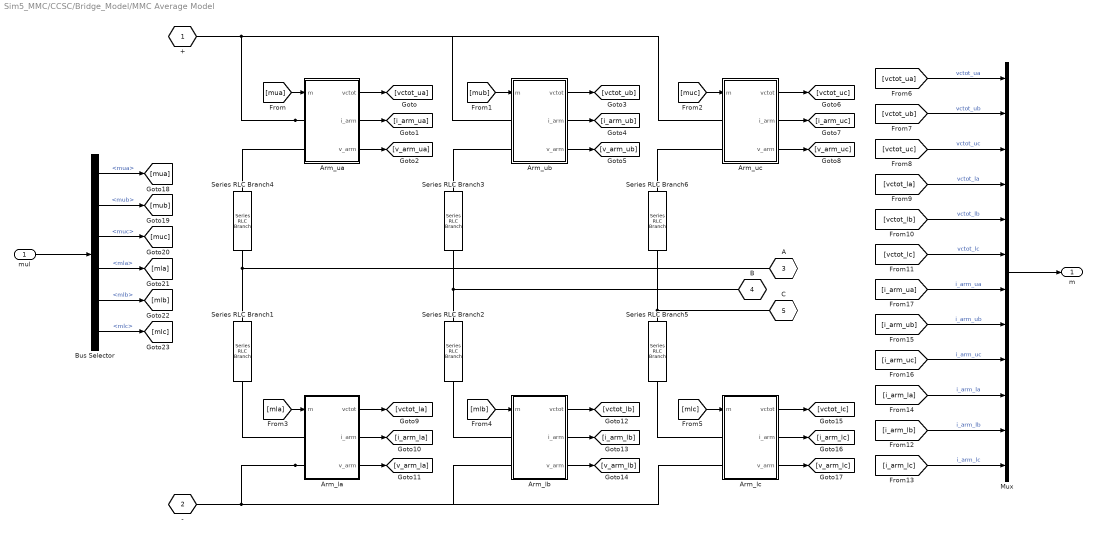
== system Sim5_MMC/CCSC/Bridge_Model/MMC Average Model ==
  mul : Inport
  Arm_la : Subsystem  mask{C_arm=Carm, Vdc=Udcn}
      mask prompts: C_arm "Arm equivalent Capacitor (F)"; Vdc "Init DC Voltage (V)"
  Arm_lb : Subsystem  mask{C_arm=Carm, Vdc=Udcn}
      mask prompts: C_arm "Arm equivalent Capacitor (F)"; Vdc "Init DC Voltage (V)"
  Arm_lc : Subsystem  mask{C_arm=Carm, Vdc=Udcn}
      mask prompts: C_arm "Arm equivalent Capacitor (F)"; Vdc "Init DC Voltage (V)"
  Arm_ua : Subsystem  mask{C_arm=Carm, Vdc=Udcn}
      mask prompts: C_arm "Arm equivalent Capacitor (F)"; Vdc "Init DC Voltage (V)"
  Arm_ub : Subsystem  mask{C_arm=Carm, Vdc=Udcn}
      mask prompts: C_arm "Arm equivalent Capacitor (F)"; Vdc "Init DC Voltage (V)"
  Arm_uc : Subsystem  mask{C_arm=Carm, Vdc=Udcn}
      mask prompts: C_arm "Arm equivalent Capacitor (F)"; Vdc "Init DC Voltage (V)"
  Bus Selector : BusSelector  OutputSignals=mua,mub,muc,mla,mlb,mlc
  Mux : Mux  Inputs=12
  Series RLC Branch{1..6} (6 alike) : powerlib/Elements/Series RLC Branch  LConnTagsString=__new0  RConnTagsString=__new0  BranchType=RL  Resistance=Rarm_pu*Zb  Inductance=Larm_pu*Lb  SetiL0=off  InitialCurrent=0  Capacitance=1e-6  Setx0=off  InitialVoltage=0  Measurements=None
  + : PMIOPort  Tag=PMCPort  Side=Right
  - : PMIOPort  Tag=PMCPort  Port=2  Side=Right
  A : PMIOPort  Tag=PMCPort  Port=3  Side=Left
  B : PMIOPort  Tag=PMCPort  Port=4  Side=Left
  C : PMIOPort  Tag=PMCPort  Port=5  Side=Left
  m : Outport
  wires:
  [mlb] -> Arm_lb/1(m)
  [mlc] -> Arm_lc/1(m)
  [mla] -> Arm_la/1(m)
  Arm_uc/1(vctot) -> [vctot_uc]
  Arm_lb/3(v_arm) -> [v_arm_lb]
  Arm_ub/3(v_arm) -> [v_arm_ub]
  Arm_ua/1(vctot) -> [vctot_ua]
  Arm_uc/2(i_arm) -> [i_arm_uc]
  Arm_lc/1(vctot) -> [vctot_lc]
  Arm_la/2(i_arm) -> [i_arm_la]
  Arm_la/1(vctot) -> [vctot_la]
  Arm_ub/2(i_arm) -> [i_arm_ub]
  Arm_lc/3(v_arm) -> [v_arm_lc]
  Arm_la/3(v_arm) -> [v_arm_la]
  [mua] -> Arm_ua/1(m)
  Arm_ub/1(vctot) -> [vctot_ub]
  Arm_lb/1(vctot) -> [vctot_lb]
  [mub] -> Arm_ub/1(m)
  Arm_uc/3(v_arm) -> [v_arm_uc]
  Arm_lb/2(i_arm) -> [i_arm_lb]
  Arm_ua/2(i_arm) -> [i_arm_ua]
  Arm_lc/2(i_arm) -> [i_arm_lc]
  [muc] -> Arm_uc/1(m)
  Arm_ua/3(v_arm) -> [v_arm_ua]
  mul/1 -> Bus Selector/1
  Bus Selector/1 -> [mua]  "<mua>"
  Bus Selector/2 -> [mub]  "<mub>"
  Bus Selector/3 -> [muc]  "<muc>"
  Bus Selector/6 -> [mlc]  "<mlc>"
  Bus Selector/5 -> [mlb]  "<mlb>"
  Bus Selector/4 -> [mla]  "<mla>"
  [vctot_lc] -> Mux/6  "vctot_lc"
  [vctot_uc] -> Mux/3  "vctot_uc"
  [i_arm_ua] -> Mux/7  "i_arm_ua"
  [i_arm_ub] -> Mux/8  "i_arm_ub"
  [vctot_lb] -> Mux/5  "vctot_lb"
  [i_arm_la] -> Mux/10  "i_arm_la"
  [vctot_ub] -> Mux/2  "vctot_ub"
  [i_arm_uc] -> Mux/9  "i_arm_uc"
  [vctot_la] -> Mux/4  "vctot_la"
  [i_arm_lb] -> Mux/11  "i_arm_lb"
  [vctot_ua] -> Mux/1  "vctot_ua"
  [i_arm_lc] -> Mux/12  "i_arm_lc"
  Mux/1 -> m/1
  connections:
  Series RLC Branch5/RConn1 -- Arm_lc/LConn1
  Arm_ua/LConn2 -- Series RLC Branch4/LConn1
  Series RLC Branch6/LConn1 -- Arm_uc/LConn2
  Series RLC Branch5/LConn1 -- Series RLC Branch6/RConn1 -- C/RConn1
  Series RLC Branch2/LConn1 -- B/RConn1 -- Series RLC Branch3/RConn1
  Arm_ub/LConn2 -- Series RLC Branch3/LConn1
  Series RLC Branch2/RConn1 -- Arm_lb/LConn1
  Series RLC Branch1/LConn1 -- Series RLC Branch4/RConn1 -- A/RConn1
  Arm_la/LConn2 -- -/RConn1 -- Arm_lc/LConn2 -- Arm_lb/LConn2
  Series RLC Branch1/RConn1 -- Arm_la/LConn1
  Arm_ua/LConn1 -- +/RConn1 -- Arm_uc/LConn1 -- Arm_ub/LConn1

== system Sim5_MMC/CCSC/Bridge_Model/Modulation Index Generation ==
  vmu_ref : Inport
  vml_ref : Inport  Port=2
  "1 -> Activer filtre notch 0 -> Désactiver filtre notch2" : Constant  Value=Udcn
  Bus Creator : BusCreator  Inputs=6
  Demux : Demux  Outputs=3
  Demux1 : Demux  Outputs=3
  Demux2 : Demux  Outputs=[3 3]
  Divide1 : Product  Inputs=/*
  Divide4 : Product  Inputs=*/
  Manual Switch : ManualSwitch  CurrentSetting=0
  Manual Switch1 : ManualSwitch
  Selector : Selector  InputPortWidth=12  IndexOptions=Index vector (dialog)  Indices=[1 2 3 4 5 6]  OutputSizes=1
  m limiter low : Saturate  UpperLimit=1  LowerLimit=0
  m limiter up : Saturate  UpperLimit=1  LowerLimit=0
  mul : Outport
  wires:
  Demux/3 -> Bus Creator/3  "muc"
  vmu_ref/1 -> Divide1/2
  Manual Switch/1 -> Divide1/1
  Bus Creator/1 -> mul/1
  Demux1/1 -> Bus Creator/4  "mla"
  Demux1/2 -> Bus Creator/5  "mlb"
  Divide4/1 -> m limiter low/1
  Demux1/3 -> Bus Creator/6  "mlc"
  Manual Switch1/1 -> Divide4/2
  Demux/2 -> Bus Creator/2  "mub"
  vml_ref/1 -> Divide4/1
  Demux/1 -> Bus Creator/1  "mua"
  m limiter up/1 -> Demux/1
  Divide1/1 -> m limiter up/1
  m limiter low/1 -> Demux1/1
  "1 -> Activer filtre notch 0 -> Désactiver filtre notch2"/1 -> Manual Switch/2, Manual Switch1/1
  Selector/1 -> Demux2/1
  [m_mmc] -> Selector/1
  Demux2/1 -> Manual Switch/1
  Demux2/2 -> Manual Switch1/2

== system Sim5_MMC/CCSC/Control loops/ pu P//Q computation ==
  v_abc_pu : Inport  PortDimensions=3
  i_abc_pu : Inport  Port=2  PortDimensions=3
  Demux : Demux  Outputs=3
      settings: DisplayOption=none
  Mux : Mux  Inputs=3
  Product1 : Product  InputSameDT=on  SaturateOnIntegerOverflow=on  OutDataTypeStr=Inherit: Same as first input
  Product3 : Product  InputSameDT=on  SaturateOnIntegerOverflow=on  OutDataTypeStr=Inherit: Same as first input
  Sum : Sum  Inputs=+-  InputSameDT=on  SaturateOnIntegerOverflow=on  OutDataTypeStr=Inherit: Same as first input
  Sum1 : Sum  Inputs=1  InputSameDT=on  SaturateOnIntegerOverflow=on  OutDataTypeStr=Inherit: Same as first input
  Sum4 : Sum  Inputs=1  InputSameDT=on  SaturateOnIntegerOverflow=on  OutDataTypeStr=Inherit: Same as first input
  Sum5 : Sum  Inputs=+-  InputSameDT=on  SaturateOnIntegerOverflow=on  OutDataTypeStr=Inherit: Same as first input
  Sum6 : Sum  Inputs=+-  InputSameDT=on  SaturateOnIntegerOverflow=on  OutDataTypeStr=Inherit: Same as first input
  pu->V : Gain  Gain=1/sqrt(3)  SaturateOnIntegerOverflow=on  OutDataTypeStr=Inherit: Same as input  ParamDataTypeStr=Inherit: Same as input
  pu->V1 : Gain  Gain=1/3  SaturateOnIntegerOverflow=on  OutDataTypeStr=Inherit: Same as input  ParamDataTypeStr=Inherit: Same as input
  pu->V2 : Gain  Gain=1/3  SaturateOnIntegerOverflow=on  OutDataTypeStr=Inherit: Same as input  ParamDataTypeStr=Inherit: Same as input
  P : Outport  VectorParamsAs1DForOutWhenUnconnected=off
  Q : Outport  Port=2  VectorParamsAs1DForOutWhenUnconnected=off
  wires:
  pu->V2/1 -> Q/1
  pu->V1/1 -> P/1
  Sum1/1 -> pu->V/1
  Product3/1 -> Sum1/1
  Product1/1 -> Sum4/1
  v_abc_pu/1 -> Product1/1, Demux/1
  i_abc_pu/1 -> Product1/2, Product3/2
  Sum4/1 -> pu->V1/1
  Demux/1 -> Sum/1, Sum6/2
  Demux/2 -> Sum/2, Sum5/1
  Demux/3 -> Sum5/2, Sum6/1
  Sum/1 -> Mux/3
  Sum5/1 -> Mux/1
  Sum6/1 -> Mux/2
  Mux/1 -> Product3/1
  pu->V/1 -> pu->V2/1  "Q"

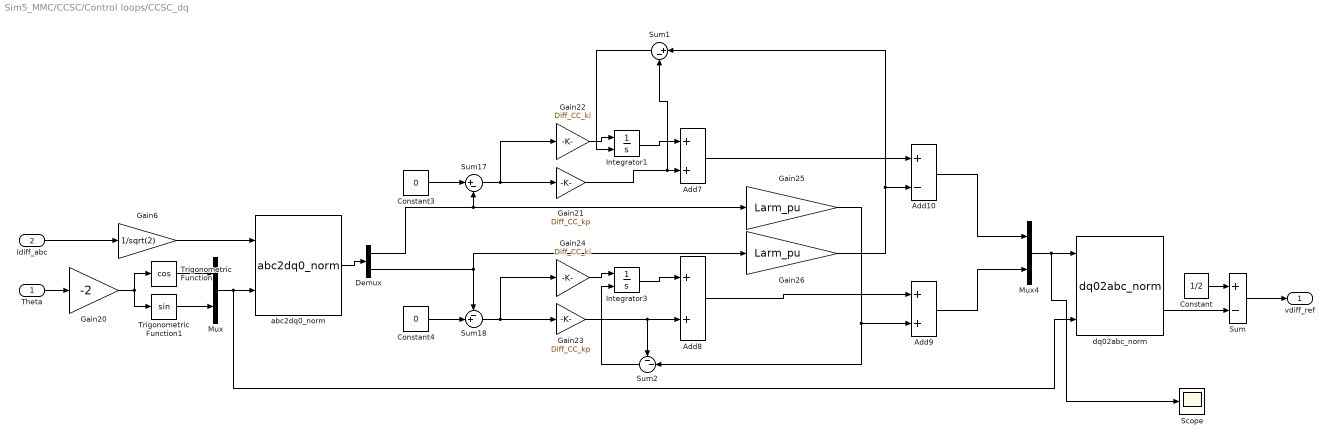
== system Sim5_MMC/CCSC/Control loops/CCSC_dq ==
  Theta : Inport
  Idiff_abc : Inport  Port=2
  Add10 : Sum  Inputs=+-
  Add7 : Sum
  Add8 : Sum
  Add9 : Sum
  Constant : Constant  Value=1/2
  Constant3 : Constant  Value=0
  Constant4 : Constant  Value=0
  Demux : Demux  Outputs=2
  Gain20 : Gain  Gain=-2
  Gain21 : Gain  Gain=Diff_CC_kp
  Gain22 : Gain  Gain=Diff_CC_ki
  Gain23 : Gain  Gain=Diff_CC_kp
  Gain24 : Gain  Gain=Diff_CC_ki
  Gain25 : Gain  Gain=Larm_pu
  Gain26 : Gain  Gain=Larm_pu
  Gain6 : Gain  Gain=1/sqrt(2)
  Integrator1 : Integrator  InitialConditionSource=external
  Integrator3 : Integrator  InitialConditionSource=external
  Mux : Mux  Inputs=2
  Mux4 : Mux  Inputs=2
  Scope : Scope
  Sum : Sum  Inputs=+-
  Sum1 : Sum  Inputs=|+-
  Sum17 : Sum  Inputs=|+-
  Sum18 : Sum  Inputs=-+|
  Sum2 : Sum  Inputs=--|
  Trigonometric Function : Trigonometry  Operator=cos
  Trigonometric Function1 : Trigonometry
  abc2dq0_norm : Control_Lib/abc2dq0_norm  referenceAxisMode=Reference axis at 90 degrees behind phase_a  baseUpdateGain=1/sqrt(3)
      settings: SourceProductName=VSC4SPS
  dq02abc_norm : Control_Lib/dq02abc_norm  referenceAxisMode=Reference axis at 90 degrees behind phase_a  baseUpdateGain=sqrt(3)
      settings: SourceProductName=VSC4SPS
  vdiff_ref : Outport
  wires:
  Theta/1 -> Gain20/1
  Constant3/1 -> Sum17/1
  Demux/2 -> Sum18/1, Gain26/1
  Add7/1 -> Add10/1
  Gain24/1 -> Integrator3/1
  Add8/1 -> Add9/1
  Idiff_abc/1 -> Gain6/1
  Sum17/1 -> Gain22/1, Gain21/1
  Gain21/1 -> Sum1/2, Add7/2
  Gain23/1 -> Sum2/1, Add8/2
  Add9/1 -> Mux4/2
  Sum18/1 -> Gain23/1, Gain24/1
  Constant4/1 -> Sum18/2
  Add10/1 -> Mux4/1
  Integrator3/1 -> Add8/1
  Mux/1 -> dq02abc_norm/3, abc2dq0_norm/2
  Gain22/1 -> Integrator1/1
  Gain25/1 -> Sum2/2, Add9/2
  Demux/1 -> Gain25/1, Sum17/2
  Integrator1/1 -> Add7/1
  Gain26/1 -> Sum1/1, Add10/2
  dq02abc_norm/2 -> Sum/2
  Gain6/1 -> abc2dq0_norm/1
  Trigonometric Function/1 -> Mux/1
  Gain20/1 -> Trigonometric Function1/1, Trigonometric Function/1
  Trigonometric Function1/1 -> Mux/2
  abc2dq0_norm/2 -> Demux/1
  Mux4/1 -> Scope/1, dq02abc_norm/1
  Sum/1 -> vdiff_ref/1
  Constant/1 -> Sum/1
  Sum1/1 -> Integrator1/2
  Sum2/1 -> Integrator3/2

== system Sim5_MMC/CCSC/Control loops/Current Limitation ==
  note: Current limitation
  Vm_dq* : Inport
  Ig_dq : Inport  Port=2
  vg_dq : Inport  Port=3
  Constant : Constant  Value=I_max_pu
  Current control : Subsystem
  Demux : Demux  Outputs=2
  Demux2 : Demux  Outputs=2
  Inverse Current control : Subsystem
  Mux : Mux  Inputs=2
  Product{,1..3} (4 alike) : Product
  Saturation Dynamic : simulink/Discontinuities/Saturation Dynamic  OutMin=[]  OutMax=[]  OutDataTypeStr=Inherit: Same as second input  OutDataType=fixdt(1, 16)  OutScaling=2^-10  DoSatur=off
  Sqrt : Sqrt  SaturateOnIntegerOverflow=on
  Sum : Sum
  Trigonometric Function : Trigonometry  Operator=atan2  NumberOfIterations=5  OutputSignalType=real
  Trigonometric Function1 : Trigonometry  Operator=cos
  Trigonometric Function2 : Trigonometry
  w_set1 : Constant
  w_set2 : Constant
  w_set3 : Constant  Value=0
  Vm_dq_sat : Outport  VectorParamsAs1DForOutWhenUnconnected=off
  wires:
  w_set3/1 -> Saturation Dynamic/3
  Constant/1 -> Saturation Dynamic/1
  Mux/1 -> Current control/1(Ig_dq0*)
  Product/1 -> Mux/1
  Demux/1 -> Product1/1, Product1/2
  Demux/2 -> Product2/1, Product2/2
  Trigonometric Function2/1 -> Product3/2
  Product2/1 -> Sum/2
  Trigonometric Function1/1 -> Product/2
  Demux2/1 -> Trigonometric Function/2
  Trigonometric Function/1 -> Trigonometric Function2/1, Trigonometric Function1/1
  Saturation Dynamic/1 -> Product/1, Product3/1
  Product1/1 -> Sum/1
  Sqrt/1 -> Saturation Dynamic/2
  Demux2/2 -> Trigonometric Function/1
  Inverse Current control/1(Is_dq*) -> Demux2/1, Demux/1
  Sum/1 -> Sqrt/1
  Product3/1 -> Mux/2
  Ig_dq/1 -> Inverse Current control/2(Ig_dq), Current control/2(Ig_dq0)
  w_set1/1 -> Inverse Current control/4(w)
  w_set2/1 -> Current control/4(w)
  vg_dq/1 -> Current control/3(vg_dq0), Inverse Current control/3(vg_dq)
  Vm_dq*/1 -> Inverse Current control/1(Vm_dq*)
  Current control/1(vm) -> Vm_dq_sat/1

== system Sim5_MMC/CCSC/Control loops/DC part: stored energy control + differential current control ==
  Wtot_ref_pu : Inport
  theta : Inport  Port=2
  vctot_up_pu : Inport  Port=3
  vctot_low_pu : Inport  Port=4
  Vdc_pu : Inport  Port=5
  pac_pu : Inport  Port=6
  idff_pu : Inport  Port=7
  vv_pu : Inport  Port=8
  Constant : Constant  Value=[0 0 0]  SampleTime=-1
  Control Wdiff : Subsystem
  "Control Wtot " : Subsystem
  Differential_current_control : Subsystem
  Sum5 : Sum
  Wdiff computation : Subsystem
  Wtot computation : Subsystem
  vdiff_pu_ref : Outport  PortDimensions=3
  wires:
  Vdc_pu/1 -> "Control Wtot "/4(Vdc_pu), Differential_current_control/1(vdc_pu)
  Wtot_ref_pu/1 -> "Control Wtot "/2(Wtot ref pu)
  "Control Wtot "/1(Idiff ref pu) -> Sum5/1
  idff_pu/1 -> Differential_current_control/2(idiff_pu)
  Sum5/1 -> Differential_current_control/3(idiff_ref_pu)
  vctot_up_pu/1 -> Wdiff computation/1(vctot u_pu), Wtot computation/1(vctot u_pu)
  vctot_low_pu/1 -> Wdiff computation/2(vctot l_pu), Wtot computation/2(vctot l_pu)
  Wdiff computation/1(Wdiff) -> Control Wdiff/1(Wdiff pu)
  Wtot computation/1(Wtot) -> "Control Wtot "/1(Wtot_pu)
  theta/1 -> Control Wdiff/3(theta)
  Constant/1 -> Control Wdiff/2(Wdiff_ref pu)
  Differential_current_control/1(Vprediff_ref_pu) -> vdiff_pu_ref/1
  pac_pu/1 -> "Control Wtot "/3(p_ac_pu)
  Control Wdiff/2(Idiff ref pu1) -> Sum5/2
  vv_pu/1 -> Control Wdiff/4(vv_pu)
